simulink model "QuarterCar_ActiveSusp_Simulink2019b"  (R2019b)
settings: Solver=ode4  StartTime=0.0  StopTime=SIM_TIME  FixedStep=STEP_SIZE  RelTol=1e-3
undefined symbols (not defined in the file): b_s, b_t, k_s, k_t, m_s, m_u
settings Model: Creator=Roberto  LastModifiedBy=Roberto
settings DataIOCC: ReturnWorkspaceOutputs=off
settings DebuggingCC: ArithmeticOperatorsInVariantConditions=warning
settings SFSimCC: CustomCodeUndefinedFunction=UseInterfaceOnly

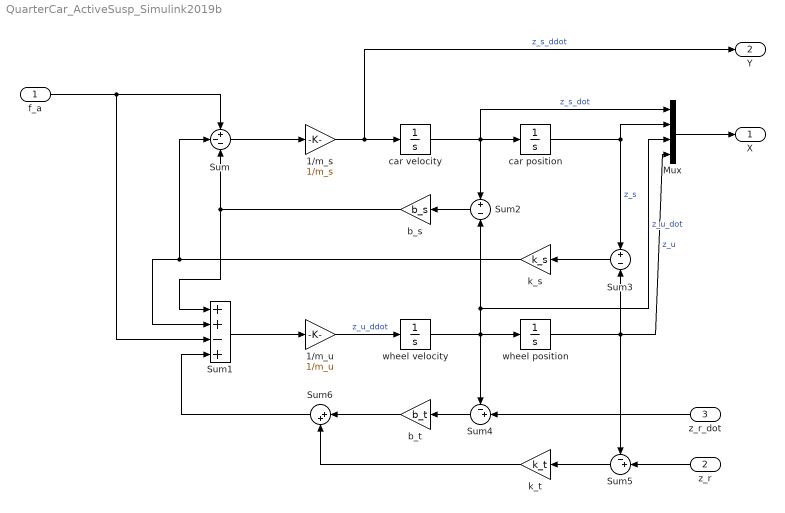
== system QuarterCar_ActiveSusp_Simulink2019b ==
  f_a : Inport
  z_r : Inport  Port=2
  z_r_dot : Inport  Port=3
  1/m_s : Gain  Gain=1/m_s
  1/m_u : Gain  Gain=1/m_u
  Mux : Mux
  Sum : Sum  Inputs=+--
  Sum1 : Sum  Inputs=++-+
  Sum2 : Sum  Inputs=+-
  Sum3 : Sum  Inputs=+-
  Sum4 : Sum  Inputs=-+|
  Sum5 : Sum  Inputs=-+|
  Sum6 : Sum  Inputs=|++
  b_s : Gain  Gain=b_s
  b_t : Gain  Gain=b_t
  car position : Integrator
  car velocity : Integrator
  k_s : Gain  Gain=k_s
  k_t : Gain  Gain=k_t
  wheel position : Integrator
  wheel velocity : Integrator
  X : Outport  VectorParamsAs1DForOutWhenUnconnected=off
  Y : Outport  Port=2  VectorParamsAs1DForOutWhenUnconnected=off
  wires:
  Mux/1 -> X/1
  Sum/1 -> 1/m_s/1
  b_s/1 -> Sum1/1, Sum/3
  k_s/1 -> Sum/2, Sum1/2
  Sum6/1 -> Sum1/4
  wheel position/1 -> Mux/4, Sum5/1, Sum3/2  "z_u"
  wheel velocity/1 -> Sum4/1, Mux/3, Sum2/2, wheel position/1  "z_u_dot"
  k_t/1 -> Sum6/2
  b_t/1 -> Sum6/1
  z_r/1 -> Sum5/2
  f_a/1 -> Sum1/3, Sum/1
  car velocity/1 -> Mux/1, Sum2/1, car position/1  "z_s_dot"
  Sum5/1 -> k_t/1
  Sum4/1 -> b_t/1
  Sum1/1 -> 1/m_u/1
  1/m_s/1 -> Y/1, car velocity/1  "z_s_ddot"
  Sum3/1 -> k_s/1
  1/m_u/1 -> wheel velocity/1  "z_u_ddot"
  Sum2/1 -> b_s/1
  car position/1 -> Mux/2, Sum3/1  "z_s"
  z_r_dot/1 -> Sum4/2
